simulink model "sampleModel1645"  (R2023a)
settings: Solver=VariableStepAuto  StartTime=0.0  StopTime=10.0  RelTol=1e-3
libraries: hdlsllib x4, simulink x2
settings Model: Creator=user1  LastModifiedBy=user1

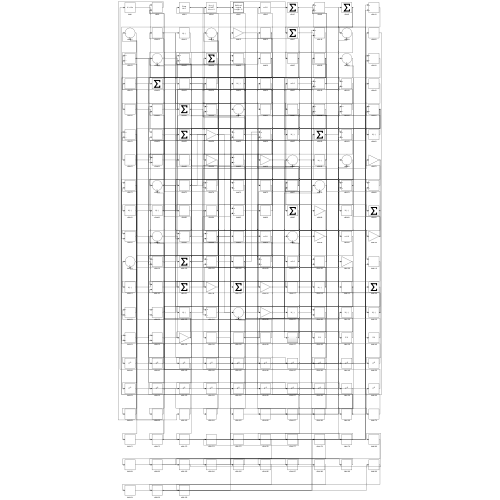
[thumbnail: Simulink's stored preview of the top-level diagram]
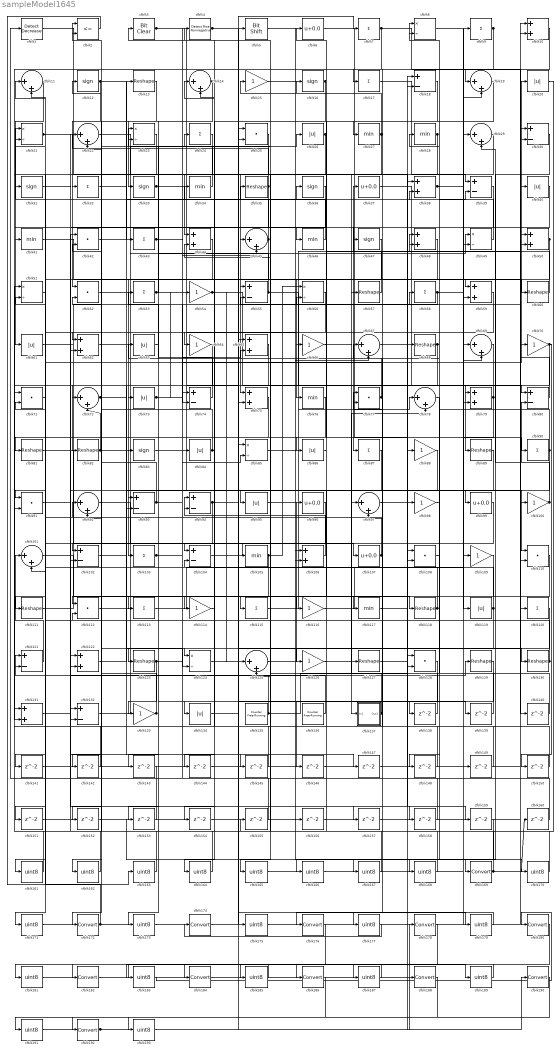
== system sampleModel1645 ==
  cfblk1 : simulink/Logic and Bit Operations/Detect Decrease  vinit=0.0  OutDataTypeStr=boolean
      settings: LibrarySourceBlock=|
      | hdlsllib/Logic and Bit
      | Operations/Detect
      | Decrease
  cfblk{10,38,44,48,50,59,62,65,75,79,106,122,131} (13 alike) : Sum
  cfblk{15,54,64,66,70,88,98,100,109,114,116,126,133} (13 alike) : Gain
  cfblk{11,14,19,22,29,45,67,69,72,78,92,97,101,125} (14 alike) : Sum  Inputs=|++
  cfblk{18,30,39,55,74,80,93..94,102,104,121,132} (12 alike) : Sum  Inputs=+-
  cfblk{7,9,17,24,32,43,53,58,87,90,103,113,115,120} (14 alike) : Sum  Inputs=+
  cfblk{27..28,34,41,46,76,105,117} (8 alike) : MinMax
  cfblk{6,37,96,99,107} (5 alike) : Bias  Bias=0.0  SaturateOnIntegerOverflow=off
  cfblk{25,42,52,71,77,91,108,110,112,128} (10 alike) : DotProduct  OutDataTypeStr=Inherit: Inherit via internal rule
  cfblk{13,35,57,60,68,81..82,89,111,118,123,127,129..130} (14 alike) : Reshape
  cfblk{20,26,40,61,63,73,84,86,95,119,134} (11 alike) : Abs  SaturateOnIntegerOverflow=off
  cfblk{12,16,31,33,36,47,83} (7 alike) : Signum
  cfblk{8,21,23,49,51,56,85,124} (8 alike) : Product  Inputs=*/  RndMeth=Zero  SaturateOnIntegerOverflow=on
  cfblk135 : hdlsllib/Sources/Counter Free-Running  NumBits=16  tsamp=-1
  cfblk136 : hdlsllib/Sources/Counter Free-Running  NumBits=16  tsamp=-1
  cfblk137 : Subsystem
      settings: LibrarySourceBlock=|
      | hdlsllib/Ports &
      | Subsystems/Subsystem
  cfblk{138..160} (23 alike) : Delay  SampleTime=1
  cfblk{161..168,170..171,173,175,177,179,181,183,185,187,189,191,193} (21 alike) : DataTypeConversion  OutDataTypeStr=uint8  SaturateOnIntegerOverflow=off  RndMeth=Floor
  cfblk{169,172,174,176,178,180,182,184,186,188,190,192} (12 alike) : DataTypeConversion  SaturateOnIntegerOverflow=off  RndMeth=Floor
  cfblk2 : RelationalOperator  Operator=<=  OutDataTypeStr=boolean  InputSameDT=off
  cfblk3 : simulink/Logic and Bit Operations/Bit Clear  iBit=0
      settings: LibrarySourceBlock=|
      | hdlsllib/Logic and Bit
      | Operations/Bit Clear
  cfblk4 : hdlsllib/Logic and Bit Operations/Detect Rise Nonnegative  vinit=0  OutDataTypeStr=boolean
  cfblk5 : hdlsllib/Logic and Bit Operations/Bit Shift  mode=Shift Left Logical  N=0
  wires:
  cfblk80/1 -> cfblk20/1
  cfblk11/1 -> cfblk61/1
  cfblk106/1 -> cfblk94/1
  cfblk37/1 -> cfblk80/1
  cfblk112/1 -> cfblk118/1
  cfblk81/1 -> cfblk104/1
  cfblk10/1 -> cfblk19/1
  cfblk83/1 -> cfblk110/1
  cfblk27/1 -> cfblk3/1, cfblk62/1, cfblk62/2
  cfblk82/1 -> cfblk26/1, cfblk39/2, cfblk72/2
  cfblk115/1 -> cfblk50/1
  cfblk127/1 -> cfblk88/1
  cfblk28/1 -> cfblk75/1, cfblk115/1, cfblk125/2
  cfblk57/1 -> cfblk6/1
  cfblk41/1 -> cfblk55/1
  cfblk35/1 -> cfblk41/1, cfblk22/1
  cfblk3/1 -> cfblk99/1, cfblk45/2
  cfblk12/1 -> cfblk52/1, cfblk47/1
  cfblk48/1 -> cfblk76/1
  cfblk23/1 -> cfblk32/1
  cfblk132/1 -> cfblk49/1
  cfblk31/1 -> cfblk46/1
  cfblk117/1 -> cfblk128/1
  cfblk95/1 -> cfblk78/1
  cfblk125/1 -> cfblk96/1
  cfblk47/1 -> cfblk103/1
  cfblk111/1 -> cfblk5/1
  cfblk113/1 -> cfblk19/2
  cfblk121/1 -> cfblk101/1
  cfblk79/1 -> cfblk73/1, cfblk106/2
  cfblk45/1 -> cfblk35/1, cfblk142/1
  cfblk52/1 -> cfblk59/1
  cfblk24/1 -> cfblk44/1
  cfblk105/1 -> cfblk56/1, cfblk152/1
  cfblk58/1 -> cfblk29/1, cfblk55/2
  cfblk63/1 -> cfblk113/1
  cfblk39/1 -> cfblk87/1
  cfblk61/1 -> cfblk10/1
  cfblk26/1 -> cfblk95/1, cfblk91/2
  cfblk13/1 -> cfblk33/1
  cfblk14/1 -> cfblk123/1, cfblk72/1
  cfblk53/1 -> cfblk23/1, cfblk85/1, cfblk106/1
  cfblk54/1 -> cfblk89/1, cfblk125/1
  cfblk103/1 -> cfblk58/1, cfblk65/2
  cfblk6/1 -> cfblk98/1
  cfblk68/1 -> cfblk48/1, cfblk93/2
  cfblk22/1 -> cfblk108/2
  cfblk118/1 -> cfblk51/2, cfblk92/2
  cfblk64/1 -> cfblk131/2
  cfblk62/1 -> cfblk9/1
  cfblk34/1 -> cfblk2/1
  cfblk70/1 -> cfblk150/1, cfblk173/1
  cfblk17/1 -> cfblk39/1
  cfblk50/1 -> cfblk79/1, cfblk86/1, cfblk91/1, cfblk153/1
  cfblk109/1 -> cfblk112/1
  cfblk130/1 -> cfblk67/1, cfblk21/2
  cfblk104/1 -> cfblk107/1
  cfblk120/1 -> cfblk172/1
  cfblk77/1 -> cfblk4/1, cfblk11/2
  cfblk55/1 -> cfblk119/1, cfblk23/2
  cfblk114/1 -> cfblk94/2
  cfblk56/1 -> cfblk111/1
  cfblk135/1 -> cfblk68/1, cfblk34/1, cfblk97/1
  cfblk96/1 -> cfblk102/1
  cfblk86/1 -> cfblk36/1
  cfblk88/1 -> cfblk132/2
  cfblk30/1 -> cfblk169/1
  cfblk94/1 -> cfblk75/2, cfblk102/2, cfblk130/1
  cfblk84/1 -> cfblk42/2, cfblk154/1
  cfblk92/1 -> cfblk127/1
  cfblk90/1 -> cfblk63/1, cfblk117/1
  cfblk7/1 -> cfblk17/1, cfblk140/1
  cfblk137/1(Out1) -> cfblk24/1, cfblk56/2
  cfblk101/1 -> cfblk114/1
  cfblk74/1 -> cfblk53/1
  cfblk59/1 -> cfblk122/2
  cfblk42/1 -> cfblk18/1
  cfblk8/1 -> cfblk109/1
  cfblk1/1 -> cfblk137/1(In1)
  cfblk100/1 -> cfblk80/2, cfblk29/2
  cfblk5/1 -> cfblk67/2
  cfblk136/1 -> cfblk121/1
  cfblk133/1 -> cfblk92/1, cfblk22/2
  cfblk36/1 -> cfblk74/2
  cfblk18/1 -> cfblk66/1
  cfblk67/1 -> cfblk128/2
  cfblk65/1 -> cfblk82/1
  cfblk60/1 -> cfblk37/1
  cfblk108/1 -> cfblk48/2
  cfblk73/1 -> cfblk70/1, cfblk54/1
  cfblk29/1 -> cfblk124/1
  cfblk9/1 -> cfblk121/2, cfblk97/2
  cfblk72/1 -> cfblk100/1, cfblk124/2
  cfblk119/1 -> cfblk126/1, cfblk14/2, cfblk162/1
  cfblk122/1 -> cfblk13/1
  cfblk25/1 -> cfblk81/1
  cfblk116/1 -> cfblk18/2
  cfblk43/1 -> cfblk93/1, cfblk60/1
  cfblk107/1 -> cfblk77/1, cfblk31/1
  cfblk49/1 -> cfblk28/1
  cfblk4/1 -> cfblk7/1, cfblk138/1
  cfblk33/1 -> cfblk38/2, cfblk45/1
  cfblk46/1 -> cfblk21/1
  cfblk44/1 -> cfblk83/1
  cfblk21/1 -> cfblk57/1, cfblk147/1
  cfblk131/1 -> cfblk129/1
  cfblk89/1 -> cfblk134/1
  cfblk123/1 -> cfblk133/1, cfblk85/2
  cfblk93/1 -> cfblk84/1, cfblk2/2
  cfblk126/1 -> cfblk78/2
  cfblk19/1 -> cfblk27/1
  cfblk87/1 -> cfblk116/1
  cfblk16/1 -> cfblk25/2, cfblk64/1
  cfblk32/1 -> cfblk43/1
  cfblk38/1 -> cfblk8/1, cfblk90/1
  cfblk138/1 -> cfblk104/2
  cfblk66/1 -> cfblk139/1
  cfblk139/1 -> cfblk44/2
  cfblk140/1 -> cfblk8/2
  cfblk99/1 -> cfblk141/1
  cfblk141/1 -> cfblk59/2
  cfblk142/1 -> cfblk51/1
  cfblk129/1 -> cfblk143/1
  cfblk143/1 -> cfblk1/1
  cfblk75/1 -> cfblk144/1
  cfblk144/1 -> cfblk110/2
  cfblk102/1 -> cfblk145/1
  cfblk145/1 -> cfblk14/1
  cfblk128/1 -> cfblk146/1
  cfblk146/1 -> cfblk79/2
  cfblk147/1 -> cfblk10/2
  cfblk98/1 -> cfblk148/1
  cfblk148/1 -> cfblk132/1
  cfblk149/1 -> cfblk77/2
  cfblk150/1 -> cfblk11/1
  cfblk76/1 -> cfblk151/1
  cfblk151/1 -> cfblk50/2
  cfblk153/1 -> cfblk112/2
  cfblk154/1 -> cfblk25/1
  cfblk20/1 -> cfblk155/1
  cfblk155/1 -> cfblk74/1
  cfblk85/1 -> cfblk156/1
  cfblk156/1 -> cfblk38/1
  cfblk91/1 -> cfblk157/1
  cfblk157/1 -> cfblk49/2
  cfblk124/1 -> cfblk158/1
  cfblk158/1 -> cfblk122/1
  cfblk97/1 -> cfblk159/1
  cfblk160/1 -> cfblk52/2
  cfblk71/1 -> cfblk161/1
  cfblk161/1 -> cfblk131/1
  cfblk162/1 -> cfblk71/1
  cfblk2/1 -> cfblk163/1
  cfblk163/1 -> cfblk71/2
  cfblk69/1 -> cfblk164/1
  cfblk164/1 -> cfblk12/1
  cfblk110/1 -> cfblk165/1
  cfblk165/1 -> cfblk69/1
  cfblk159/1 -> cfblk166/1
  cfblk166/1 -> cfblk69/2
  cfblk15/1 -> cfblk167/1
  cfblk167/1 -> cfblk42/1
  cfblk78/1 -> cfblk168/1
  cfblk168/1 -> cfblk15/1
  cfblk169/1 -> cfblk160/1, cfblk65/1, cfblk16/1
  cfblk152/1 -> cfblk170/1
  cfblk170/1 -> cfblk30/1
  cfblk51/1 -> cfblk171/1
  cfblk171/1 -> cfblk30/2
  cfblk172/1 -> cfblk149/1, cfblk101/2
  cfblk173/1 -> cfblk120/1
  cfblk134/1 -> cfblk175/1
  cfblk175/1 -> cfblk40/1
  cfblk40/1 -> cfblk177/1
  cfblk177/1 -> cfblk174/1
  cfblk174/1 -> cfblk179/1
  cfblk179/1 -> cfblk176/1
  cfblk176/1 -> cfblk181/1
  cfblk181/1 -> cfblk178/1
  cfblk178/1 -> cfblk183/1
  cfblk183/1 -> cfblk180/1
  cfblk180/1 -> cfblk185/1
  cfblk185/1 -> cfblk182/1
  cfblk182/1 -> cfblk187/1
  cfblk187/1 -> cfblk184/1
  cfblk184/1 -> cfblk189/1
  cfblk189/1 -> cfblk186/1
  cfblk190/1 -> cfblk192/1
  cfblk186/1 -> cfblk191/1
  cfblk191/1 -> cfblk188/1
  cfblk192/1 -> cfblk108/1, cfblk105/1
  cfblk188/1 -> cfblk193/1
  cfblk193/1 -> cfblk190/1

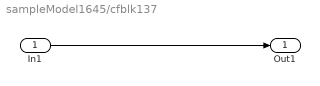
== system sampleModel1645/cfblk137 ==
  In1 : Inport
  Out1 : Outport
  wires:
  In1/1 -> Out1/1
